simulink model "force_control"  (R2022b)
settings: Solver=VariableStepAuto  StartTime=0.0  StopTime=10.0  RelTol=1e-3
values from neighbouring files (symbols this model uses):
  a = [a(1),a(2),a(3)]    [final_test_pd_control.m]    (also in force_control.m; getBCG.m = [a1;a2;a3]; governorning_equation.m = [a1;a2]; motion_equation.m = dhs(:,3))
  iL = 11*[1 1 1]'    [final_test_pd_control.m]    (also in force_control.m = IL*[1 1 1]'; getBCG.m = [iL1 iL2 iL3]; pd_control.m = IL*[1 1 1]')
  im = 0.03*[1 1 1]'    [final_test_pd_control.m]    (also in force_control.m = IM*[1 1 1]'; getBCG.m = [im1 im2 im3]; pd_control.m = IM*[1 1 1]')
  K_D = 200    [final_test_pd_control.m]    (also in force_control.m = K_D; pd_control.m = K_D)
  K_P = 450    [final_test_pd_control.m]    (also in force_control.m = K_P; pd_control.m = K_P)
  kr = 110*[1 1 1]'    [final_test_pd_control.m]    (also in force_control.m = KR*[1 1 1]'; getBCG.m = [kr1 kr2 kr3]; governorning_equation.m = [kr1 kr2]; motion_equation.m = [kr(1) kr(2) kr(3) kr(4) kr(5)])
  l = 0.5*a'    [final_test_pd_control.m]    (also in force_control.m = L *a'; pd_control.m = L *a')
  mL = 50*[1 1 1]'    [final_test_pd_control.m]    (also in force_control.m = ML*[1 1 1]'; pd_control.m = ML*[1 1 1]')
  mm = 50*[1 1 1]'    [final_test_pd_control.m]    (also in force_control.m = MM*[1 1 1]'; getBCG.m = [mm1 mm2 mm3]; governorning_equation.m = [mm1 mm2]; motion_equation.m = [mm(1) mm(2) mm(3) mm(4) mm(5)])
  qi = [0.5;0.5;0.5]    [final_test_pd_control.m]    (also in force_control.m; impedance_entrance.m = [q1 q2]; pd_control.m)
  Ts = 0.02    [final_test_pd_control.m]    (also in force_control.m; pd_control.m)
  xd = [1 1 0]    [final_test_pd_control.m]    (also in force_control.m; impedance_entrance.m = [xd1 xd2]; pd_control.m = xd)
settings Model: Creator=amarn  LastModifiedBy=sherrysajan
settings DataIOCC: SaveFormat=Array  SaveOutput=off  ReturnWorkspaceOutputsName=ans
settings OptimizationCC: BlockReduction=off  DefaultParameterBehavior=Inlined  BufferReuse=off  ReuseModelBlockBuffer=on

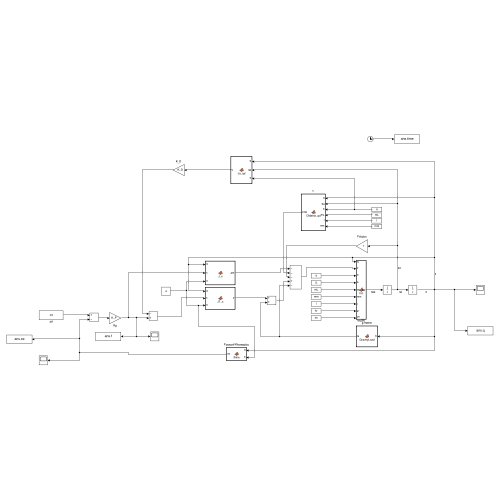
[thumbnail: Simulink's stored preview of the top-level diagram]
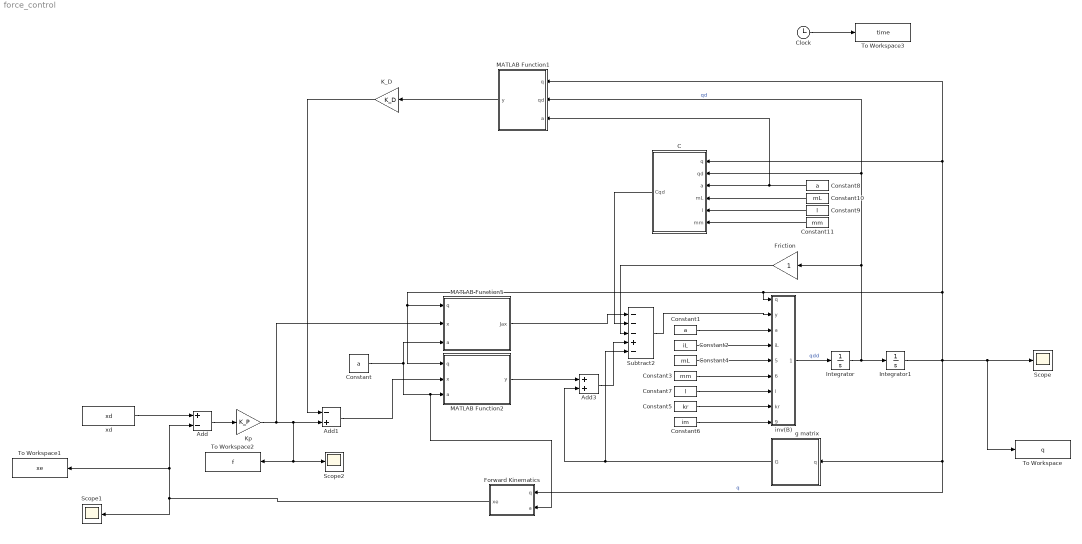
== system force_control ==
  Add : Sum  Inputs=+-
  Add1 : Sum  Inputs=-+
  Add3 : Sum
  C : MATLAB Function  TreatAsAtomicUnit=on
  Clock : Clock
  Constant : Constant  Value=a  SampleTime=Ts
  Constant1 : Constant  Value=a  SampleTime=Ts
  Constant10 : Constant  Value=mL  SampleTime=Ts
  Constant11 : Constant  Value=mm  SampleTime=Ts
  Constant2 : Constant  Value=iL  SampleTime=Ts
  Constant3 : Constant  Value=mm  SampleTime=Ts
  Constant4 : Constant  Value=mL  SampleTime=Ts
  Constant5 : Constant  Value=kr  SampleTime=Ts
  Constant6 : Constant  Value=im  SampleTime=Ts
  Constant7 : Constant  Value=l  SampleTime=Ts
  Constant8 : Constant  Value=a  SampleTime=Ts
  Constant9 : Constant  Value=l  SampleTime=Ts
  Forward Kinematics : MATLAB Function  TreatAsAtomicUnit=on
  Friction : Gain
  Integrator : Integrator  InitialCondition=[0; 0;0]
  Integrator1 : Integrator  InitialCondition=qi
  K_D : Gain  Gain=K_D
  Kp : Gain  Gain=K_P
  MATLAB Function1 : MATLAB Function  TreatAsAtomicUnit=on
  MATLAB Function2 : MATLAB Function  TreatAsAtomicUnit=on
  MATLAB Function5 : MATLAB Function  TreatAsAtomicUnit=on
  Scope : Scope
  Scope1 : Scope
  Scope2 : Scope
  Subtract2 : Sum  Inputs=---+-
  To Workspace : ToWorkspace  VariableName=q  SampleTime=Ts
      settings: Save2DSignal=2-D array (concatenate along first dimension)
  To Workspace1 : ToWorkspace  VariableName=xe  SampleTime=Ts
      settings: Save2DSignal=2-D array (concatenate along first dimension)
  To Workspace2 : ToWorkspace  VariableName=f  SampleTime=Ts
      settings: Save2DSignal=2-D array (concatenate along first dimension)
  To Workspace3 : ToWorkspace  VariableName=time  SampleTime=Ts
      settings: Save2DSignal=2-D array (concatenate along first dimension)
  g matrix : MATLAB Function  TreatAsAtomicUnit=on
  inv(B) : MATLAB Function  TreatAsAtomicUnit=on
  xd : Constant  Value=xd  SampleTime=Ts
  wires:
  Constant11/1 -> C/6(mm)
  Add/1 -> Kp/1
  Constant7/1 -> inv(B)/7(l)
  Subtract2/1 -> inv(B)/2(y)
  g matrix/1(G) -> Subtract2/5, Add3/2
  Constant8/1 -> MATLAB Function1/3(a), C/3(a)
  Constant3/1 -> inv(B)/6(mm)
  Kp/1 -> MATLAB Function5/2(x), To Workspace2/1, Scope2/1, Add1/2
  Constant/1 -> MATLAB Function5/3(a), Forward Kinematics/2(a), MATLAB Function2/3(a)
  K_D/1 -> Add1/1
  inv(B)/1(By) -> Integrator/1  "qdd"
  MATLAB Function2/1(y) -> Add3/1
  Constant2/1 -> inv(B)/4(iL)
  MATLAB Function5/1(Jax) -> Subtract2/1
  Add1/1 -> MATLAB Function2/2(x)
  MATLAB Function1/1(y) -> K_D/1
  Add3/1 -> Subtract2/4
  Constant1/1 -> inv(B)/3(a)
  Constant5/1 -> inv(B)/8(kr)
  Constant9/1 -> C/5(l)
  Friction/1 -> Subtract2/3
  Forward Kinematics/1(xe) -> Scope1/1, To Workspace1/1, Add/2
  Integrator1/1 -> MATLAB Function1/1(q), C/1(q), inv(B)/1(q), MATLAB Function2/1(q), MATLAB Function5/1(q), To Workspace/1, Scope/1, Forward Kinematics/1(q), g matrix/1(q)  "q"
  Integrator/1 -> MATLAB Function1/2(qd), C/2(qd), Friction/1, Integrator1/1  "qd"
  Constant10/1 -> C/4(mL)
  xd/1 -> Add/1
  Constant6/1 -> inv(B)/9(im)
  C/1(Cqd) -> Subtract2/2
  Constant4/1 -> inv(B)/5(mL)
  Clock/1 -> To Workspace3/1

== matlab function force_control/MATLAB Function1 ==
  data: q input; qd input; y output; a input
function y = Ja_qd(q,qd,a)
Ja = zeros(3,3);
Ja(1:2,3) = [-a(3)*sin(q(1)+q(2)+q(3));a(3)*cos(q(1)+q(2)+q(3))]; % [-a(3)*S123 ; a(3)*C123]
Ja(1:2,2) = [-a(2)*sin(q(1)+q(2));a(2)*cos(q(1)+q(2))] + Ja(1:2,3);% [-a(2)*S12-a(3)*S123 ;a(2)*C12+a(3)*C123]
Ja(1:2,1) = [-a(1)*sin(q(1));a(1)*cos(q(1))]+Ja(1:2,2);          % [-a(1)*s_1 - a(2)*S12 - a(3)*S123 ;a(1)*c_1 + a(2)*C12 + a(3)*C123]
Ja(3,:) = [0 0 0];

y = Ja*qd;

== matlab function force_control/MATLAB Function5 ==
  data: q input; Jax output; x input; a input
function Jax = J_x(q,x,a)

Ja = zeros(3,3);
Ja(1:2,3) = [-a(3)*sin(q(1)+q(2)+q(3));a(3)*cos(q(1)+q(2)+q(3))] ;   % [-a(3)*S123 ; a(3)*C123]
Ja(1:2,2) = [-a(2)*sin(q(1)+q(2));a(2)*cos(q(1)+q(2))] + Ja(1:2,3) ; % [-a(2)*S12-a(3)*S123 ;a(2)*C12+a(3)*C123]
Ja(1:2,1) = [-a(1)*sin(q(1));a(1)*cos(q(1))]+Ja(1:2,2)  ; % [-a(1)*s_1 - a(2)*S12 - a(3)*S123 ;a(1)*c_1 + a(2)*C12 + a(3)*C123]
Ja(3,:) = [0 0 0];
Jax = Ja*x;

== matlab function force_control/inv(B) ==
  data: q input; By output; y input; a input; iL input; mL input; mm input; l input; kr input; im input
function By = fcn(q,y,a,iL,mL,mm,l,kr,im)

if nargin==1
    q = [0.5*pi;0.5*pi,0.5*pi];
end
 c = @(x) cos(x);
 s = @(x) sin(x);

B11 = iL(1) + iL(2) + iL(3) + im(2) + im(3) + a(1)^2*mL(2) + a(1)^2*mL(3)...
    + a(2)^2*mL(3) + a(1)^2*mm(2) + a(1)^2*mm(3) + a(2)^2*mm(3) + im(1)*kr(1)^2 ...
    + l(1)^2*mL(1) + l(2)^2*mL(2) + l(3)^2*mL(3) + 2*a(1)*l(3)*mL(3)*c(q(2)...
    + q(3)) + 2*a(1)*a(2)*mL(3)*c(q(2)) + 2*a(1)*a(2)*mm(3)*c(q(2)) ...
    + 2*a(1)*l(2)*mL(2)*c(q(2)) + 2*a(2)*l(3)*mL(3)*c(q(3));

B12 = iL(2) + iL(3) + im(3) + im(2)*kr(2) + a(2)^2*mL(3) + a(2)^2*mm(3) ...
    + l(2)^2*mL(2) + l(3)^2*mL(3) + a(1)*l(3)*mL(3)*c(q(2) + q(3)) ...
    + a(1)*a(2)*mL(3)*c(q(2)) + a(1)*a(2)*mm(3)*c(q(2)) ...
    + a(1)*l(2)*mL(2)*c(q(2)) + 2*a(2)*l(3)*mL(3)*c(q(3));

B13 = iL(3) + im(3)*kr(3);
B21 = iL(2) + iL(3) + im(3) + im(2)*kr(2) + a(2)^2*mL(3) + a(2)^2*mm(3)...
    + l(2)^2*mL(2) + l(3)^2*mL(3) + a(1)*l(3)*mL(3)*c(q(2) + q(3)) ...
    + a(1)*a(2)*mL(3)*c(q(2)) + a(1)*a(2)*mm(3)*c(q(2)) ...
    + a(1)*l(2)*mL(2)*c(q(2)) + 2*a(2)*l(3)*mL(3)*c(q(3));

B22 = iL(2) + iL(3) + im(3) + a(2)^2*mL(3) + a(2)^2*mm(3) + im(2)*kr(2)^2 ...
    + l(2)^2*mL(2) + l(3)^2*mL(3) + 2*a(2)*l(3)*mL(3)*c(q(3));

B23 = iL(3) + im(3)*kr(3);
B31 = iL(3) + im(3)*kr(3);
B32 = iL(3) + im(3)*kr(3);
B33 = im(3)*kr(3)^2 + iL(3);

B = [B11 B12 B13;B21 B22 B23;B31 B32 B33];

By = inv(B)*y;

== matlab function force_control/C ==
  data: q input; Cqd output; qd input; a input; mL input; l input; mm input
function Cqd = CMatrix_qd(q,qd,a,mL,l,mm)

 c = @(x) cos(x);
 s = @(x) sin(x);


C11 = - a(1)*qd(2)*(a(2)*mL(3)*s(q(2)) + a(2)*mm(3)*s(q(2)) ...
    + l(2)*mL(2)*s(q(2)) + l(3)*mL(3)*s(q(2) + q(3))) ...
    - l(3)*mL(3)*qd(3)*(a(1)*s(q(2) + q(3)) + a(2)*s(q(3)));

C12 = - a(1)*qd(1)*(a(2)*mL(3)*s(q(2)) + a(2)*mm(3)*s(q(2)) ...
    + l(2)*mL(2)*s(q(2)) + l(3)*mL(3)*s(q(2) + q(3))) ...
    - a(1)*qd(2)*(a(2)*mL(3)*s(q(2)) + a(2)*mm(3)*s(q(2)) ...
    + l(2)*mL(2)*s(q(2)) + l(3)*mL(3)*s(q(2) + q(3))) ...
    - (l(3)*mL(3)*qd(3)*(a(1)*s(q(2) + q(3)) + 2*a(2)*s(q(3))))/2;

C13 = - qd(1)*(a(1)*l(3)*mL(3)*s(q(2) + q(3)) + a(2)*l(3)*mL(3)*s(q(3))) ...
    - qd(2)*((a(1)*l(3)*mL(3)*s(q(2) + q(3)))/2 + a(2)*l(3)*mL(3)*s(q(3)));

C21= a(1)*qd(1)*(a(2)*mL(3)*s(q(2)) + a(2)*mm(3)*s(q(2)) ...
    + l(2)*mL(2)*s(q(2)) + l(3)*mL(3)*s(q(2) + q(3))) ...
    - (l(3)*mL(3)*qd(3)*(a(1)*s(q(2) + q(3)) + 2*a(2)*s(q(3))))/2;

C22 = -a(2)*l(3)*mL(3)*qd(3)*s(q(3));

C23 = - qd(1)*((a(1)*l(3)*mL(3)*s(q(2) + q(3)))/2 + a(2)*l(3)*mL(3)*s(q(3))) ...
    - a(2)*l(3)*mL(3)*qd(2)*s(q(3));

C31 = qd(1)*(a(1)*l(3)*mL(3)*s(q(2) + q(3)) + a(2)*l(3)*mL(3)*s(q(3))) ...
    + qd(2)*((a(1)*l(3)*mL(3)*s(q(2) + q(3)))/2 + a(2)*l(3)*mL(3)*s(q(3)));
C32 = qd(1)*((a(1)*l(3)*mL(3)*s(q(2) + q(3)))/2 + a(2)*l(3)*mL(3)*s(q(3))) ...
    + a(2)*l(3)*mL(3)*qd(2)*s(q(3));
C33 = 0;


C = [C11 C12 C13; C21 C22 C23;C31 C32 C33];
Cqd = C*qd;

== matlab function force_control/g matrix ==
  data: q input; G output
function G = GravityLoad(q)


G = [0 ;0 ;0];

== matlab function force_control/Forward Kinematics ==
  data: q input; xe output; a input
function xe = fkine(q,a)

xe = [a(1)*cos(q(1))+a(2)*cos(q(1)+q(2))+a(3)*cos(q(1)+q(2)+q(3)) a(1)*sin(q(1))+a(2)*sin(q(1)+q(2))+a(3)*sin(q(1)+q(2)+q(3)) 0];

== matlab function force_control/MATLAB Function2 ==
  data: q input; y output; x input; a input
function y = JT_x(q,x,a)

Ja = zeros(3,3);
Ja(1:2,3) = [-a(3)*sin(q(1)+q(2)+q(3));a(3)*cos(q(1)+q(2)+q(3))];    % [-a(3)*S123 ; a(3)*C123]
Ja(1:2,2) = [-a(2)*sin(q(1)+q(2));      a(2)*cos(q(1)+q(2))] + Ja(1:2,3);  % [-a(2)*S12-a(3)*S123 ;a(2)*C12+a(3)*C123]
Ja(1:2,1) = [-a(1)*sin(q(1));           a(1)*cos(q(1))]+Ja(1:2,2) ;             % [-a(1)*s_1 - a(2)*S12 - a(3)*S123 ;a(1)*c_1 + a(2)*C12 + a(3)*C123]
Ja(3,:) = [0 0 0];
y = Ja'*x;
